simulink model "Super12"  (Simulink 5.0)
settings: Solver=ode45  StartTime=0.0  StopTime=10.0  RelTol=1e-3
settings Model: Creator=scaife  LastModifiedBy=scaife  ExtModeAutoUpdateStatusClock=off

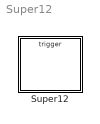
== system Super12 ==
  Super12 : Stateflow chart

== stateflow chart Super12 ==
  state A
    state A1
    (default) -> A1
  state B
    state B1
  (default) -> A
  A1 -> B1 : E
  B1 -> A1 : F
  events: E input EITHER_EDGE_EVENT; F input EITHER_EDGE_EVENT
